simulink model "SIM_3DoF"  (R2024b)
settings: Solver=VariableStepAuto  StartTime=0.0  StopTime=300  RelTol=1e-6
values from neighbouring files (symbols this model uses):
  CL_zero = 0    [my_parameter_search.m]
  delta_maneuver = 1    [my_parameter_search.m]    (also in run_3DoF_SIM_SR22.m = 10; run_3DoF_SIM_SR22_Controller_Test.m = 0)
  deltaE = op_point.Inputs(1).u    [my_parameter_search.m]    (also in run_3DoF_SIM.m = -10; run_3DoF_SIM_SR22.m; run_3DoF_SIM_SR22_Controller_Test.m)
  gravity = 9.807    [run_3DoF_SIM.m]
  J = 30    [run_3DoF_SIM.m]
  M = M - 200    [my_parameter_search.m]
  p_maneuver = 1.5    [my_parameter_search.m]    (also in run_3DoF_SIM_SR22.m; run_3DoF_SIM_SR22_Controller_Test.m)
  rate_maneuver = 7    [my_parameter_search.m]    (also in run_3DoF_SIM_SR22.m; run_3DoF_SIM_SR22_Controller_Test.m)
  states_init = [0 op_point.States.x(2) op_point.States.x(3) op_point.States.x(4) 0 0]    [my_parameter_search.m]    (also in run_3DoF_SIM.m = [0 5000 0 80 0 0]; run_3DoF_SIM_SR22.m; run_3DoF_SIM_SR22_Controller_Test.m)
  t_maneuver = 0    [my_parameter_search.m]    (also in run_3DoF_SIM_SR22.m = 100; run_3DoF_SIM_SR22_Controller_Test.m)
  throttle = op_point.Inputs(2).u    [my_parameter_search.m]    (also in run_3DoF_SIM.m = 0.65; run_3DoF_SIM_SR22.m; run_3DoF_SIM_SR22_Controller_Test.m)
undefined symbols (not defined in the file or in its folder): CD_alpha, CL_alpha, CL_elev, CLEH_alpha, Cm_zero, Cw, down_wash, Sh, Sw, xa, xt
libraries: simulink_extras x7, aerolibatmos2 x2, slpidlib x2
(part 1 of 2)
settings Model: Creator=diego  LastModifiedBy=nicom

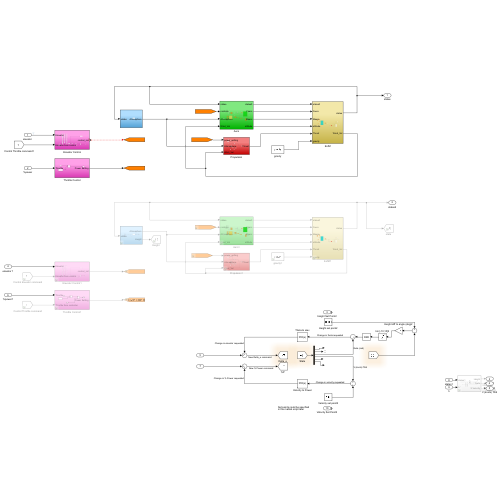
[thumbnail: Simulink's stored preview of the top-level diagram]
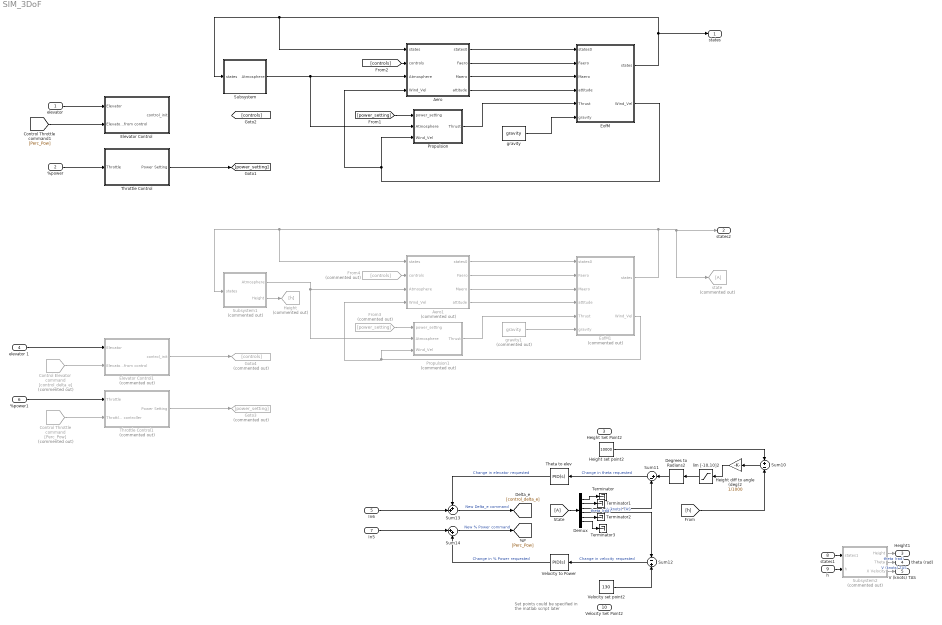
== system SIM_3DoF ==
  note: Set points could be specified in the matlab script later
  "elevator " : Inport
  %power : Inport  Port=2
  Height Set Point2 : Inport  Port=3
  elevator 1 : Inport  Port=4
  In6 : Inport  Port=5
  %power1 : Inport  Port=6
  In5 : Inport  Port=7
  states1 : Inport  Port=8
  h : Inport  Port=9
  Velocity Set Point2 : Inport  Port=10
  Aero : Subsystem
  Aero1 : Subsystem  Commented=on
  Control Elevator command : From  Commented=on  GotoTag=control_delta_e
  Control Throttle command : From  Commented=on  GotoTag=Perc_Pow
  Degrees to Radians2 : simulink_extras/Transformations/Degrees to Radians
  Demux : Demux  Outputs=6
  Elevator Control : Subsystem
  Elevator Control1 : Subsystem  Commented=on
  EofM : Subsystem
  EofM1 : Subsystem  Commented=on
  From3 : From  Commented=on  GotoTag=power_setting
  From4 : From  Commented=on  GotoTag=controls
  Goto3 : Goto  Commented=on  GotoTag=power_setting
  Goto4 : Goto  Commented=on  GotoTag=controls
  Height : Goto  Commented=on  GotoTag=h
  Height diff to angle (deg)2 : Gain  Gain=1/1000
  Height set point2 : Constant  Value=10000
  Propulsion : Subsystem
  Propulsion1 : Subsystem  Commented=on
  State : From
  Subsystem : Subsystem
  Subsystem1 : Subsystem  Commented=on
  Subsystem2 : Subsystem  Commented=on
  Sum10 : Sum  Inputs=+|-
  Sum11 : Sum  Inputs=|+-
  Sum12 : Sum  Inputs=-|+
  Sum13 : Sum  Inputs=++|
  Sum14 : Sum  Inputs=|++
  Terminator{,1..3} (4 alike) : Terminator
  Theta to elev : slpidlib/PID Controller  Controller=PID  Form=Parallel  TimeDomain=Continuous-time  UseExternalTs=off  SampleTime=-1  IntegratorMethod=Forward Euler  FilterMethod=Forward Euler  ControllerParametersSource=internal  P=1  I=1  UseKiTs=off  D=0  UseExternalDerivativeSource=off  N=100  UseFilter=on  TunerSelectOption=Transfer Function Based (PID Tuner App)  InitialConditionSource=internal  InitialConditionForIntegrator=0  InitialConditionForFilter=0  DifferentiatorICPrevScaledInput=0  ExternalReset=none  TrackingMode=off  Kt=1  LimitOutput=off  SatLimitsSource=internal  UpperSaturationLimit=inf  LowerSaturationLimit=-inf  LinearizeAsGain=on  AntiWindupMode=none  Kb=1  LimitIntegrator=off  UpperIntegratorSaturationLimit=inf  LowerIntegratorSaturationLimit=-inf  POutMin=[]  POutMax=[]  IOutMin=[]  IOutMax=[]  DOutMin=[]  DOutMax=[]  NOutMin=[]  NOutMax=[]  SumOutMin=[]  SumOutMax=[]  SaturationOutMin=[]  SaturationOutMax=[]  PParamMin=[]  PParamMax=[]  IParamMin=[]  IParamMax=[]  DParamMin=[]  DParamMax=[]  NParamMin=[]  NParamMax=[]  KbParamMin=[]  KbParamMax=[]  KtParamMin=[]  KtParamMax=[]  KbOutMin=[]  KbOutMax=[]  KtOutMin=[]  KtOutMax=[]  IntegratorOutMin=[]  IntegratorOutMax=[]  FilterOutMin=[]  FilterOutMax=[]  SumI1OutMin=[]  SumI1OutMax=[]  SumI2OutMin=[]  SumI2OutMax=[]  SumI3OutMin=[]  SumI3OutMax=[]  SumI4OutMin=[]  SumI4OutMax=[]  SumDOutMin=[]  SumDOutMax=[]  DifferentiatorOutMin=[]  DifferentiatorOutMax=[]  FilterDiffOutCoefMin=[]  FilterDiffOutCoefMax=[]  ReciprocalOutMin=[]  ReciprocalOutMax=[]  SumDenOutMin=[]  SumDenOutMax=[]  SumNumOutMin=[]  SumNumOutMax=[]  DivideOutMin=[]  DivideOutMax=[]  UdiffTsProdOutMin=[]  UdiffTsProdOutMax=[]  NTsProdOutMin=[]  NTsProdOutMax=[]  UintegralTsProdOutMin=[]  UintegralTsProdOutMax=[]  UngainTsProdOutMin=[]  UngainTsProdOutMax=[]  ClampingZeroOutDataTypeStr=Inherit: Inherit via back propagation  ClampingZeroOutMin=[]  ClampingZeroOutMax=[]  FilterDenConstantOutDataTypeStr=Inherit: Inherit via back propagation  FilterDenConstantOutMin=[]  FilterDenConstantOutMax=[]  PCopyOutDataTypeStr=Inherit: Inherit via back propagation  PCopyOutMin=[]  PCopyOutMax=[]  NCopyOutDataTypeStr=Inherit: Inherit via back propagation  NCopyOutMin=[]  NCopyOutMax=[]  IntegratorContinuousStateAttributes=''  IntegratorStateMustResolveToSignalObject=off  IntegratorRTWStateStorageClass=Auto  FilterContinuousStateAttributes=''  FilterStateMustResolveToSignalObject=off  FilterRTWStateStorageClass=Auto  ParallelPVariant=InternalParameters  IdealPVariant=Disabled  IVariant=InternalParameters  DVariant=InternalParameters  IntegratorVariant=Continuous  SatVariant=Disabled  AWVariant=Passthrough  PCopyVariant=Disabled  TRVariant=Disabled  FdbkBlocksVariant=Forward  IdealPFdbkVariant=Disabled  SatFdbkVariant=Disabled  DerivativeFilterVariant=ContFilter  NVariant=InternalParameters  NCopyVariant=Disabled  FilterICVariant=InternalICsFilter  IntegratorICVariant=InternalICs  ExternalResetVariant=Disabled  TRSumVariant=Passthrough  SumFdbkVariant=Disabled  SumVariant=Sum_PID  TsampFilterVariant=InternalTs  TsampNgainVariant=Passthrough  TsampIntegralVariant=Disabled_SignalSpec  ExternalSaturationOutDataTypeStr=Inherit: Same as second input  DerivativeSourceVariant=ErrorSignal  PreIntVariant=InternalPreInt
  Throttle Control : Subsystem
  Throttle Control1 : Subsystem  Commented=on
  Velocity set point2 : Constant  Value=130
  Velocity to Power : slpidlib/PID Controller  Controller=PID  Form=Parallel  TimeDomain=Continuous-time  UseExternalTs=off  SampleTime=-1  IntegratorMethod=Forward Euler  FilterMethod=Forward Euler  ControllerParametersSource=internal  P=1  I=1  UseKiTs=off  D=0  UseExternalDerivativeSource=off  N=100  UseFilter=on  TunerSelectOption=Transfer Function Based (PID Tuner App)  InitialConditionSource=internal  InitialConditionForIntegrator=0  InitialConditionForFilter=0  DifferentiatorICPrevScaledInput=0  ExternalReset=none  TrackingMode=off  Kt=1  LimitOutput=off  SatLimitsSource=internal  UpperSaturationLimit=inf  LowerSaturationLimit=-inf  LinearizeAsGain=on  AntiWindupMode=none  Kb=1  LimitIntegrator=off  UpperIntegratorSaturationLimit=inf  LowerIntegratorSaturationLimit=-inf  POutMin=[]  POutMax=[]  IOutMin=[]  IOutMax=[]  DOutMin=[]  DOutMax=[]  NOutMin=[]  NOutMax=[]  SumOutMin=[]  SumOutMax=[]  SaturationOutMin=[]  SaturationOutMax=[]  PParamMin=[]  PParamMax=[]  IParamMin=[]  IParamMax=[]  DParamMin=[]  DParamMax=[]  NParamMin=[]  NParamMax=[]  KbParamMin=[]  KbParamMax=[]  KtParamMin=[]  KtParamMax=[]  KbOutMin=[]  KbOutMax=[]  KtOutMin=[]  KtOutMax=[]  IntegratorOutMin=[]  IntegratorOutMax=[]  FilterOutMin=[]  FilterOutMax=[]  SumI1OutMin=[]  SumI1OutMax=[]  SumI2OutMin=[]  SumI2OutMax=[]  SumI3OutMin=[]  SumI3OutMax=[]  SumI4OutMin=[]  SumI4OutMax=[]  SumDOutMin=[]  SumDOutMax=[]  DifferentiatorOutMin=[]  DifferentiatorOutMax=[]  FilterDiffOutCoefMin=[]  FilterDiffOutCoefMax=[]  ReciprocalOutMin=[]  ReciprocalOutMax=[]  SumDenOutMin=[]  SumDenOutMax=[]  SumNumOutMin=[]  SumNumOutMax=[]  DivideOutMin=[]  DivideOutMax=[]  UdiffTsProdOutMin=[]  UdiffTsProdOutMax=[]  NTsProdOutMin=[]  NTsProdOutMax=[]  UintegralTsProdOutMin=[]  UintegralTsProdOutMax=[]  UngainTsProdOutMin=[]  UngainTsProdOutMax=[]  ClampingZeroOutDataTypeStr=Inherit: Inherit via back propagation  ClampingZeroOutMin=[]  ClampingZeroOutMax=[]  FilterDenConstantOutDataTypeStr=Inherit: Inherit via back propagation  FilterDenConstantOutMin=[]  FilterDenConstantOutMax=[]  PCopyOutDataTypeStr=Inherit: Inherit via back propagation  PCopyOutMin=[]  PCopyOutMax=[]  NCopyOutDataTypeStr=Inherit: Inherit via back propagation  NCopyOutMin=[]  NCopyOutMax=[]  IntegratorContinuousStateAttributes=''  IntegratorStateMustResolveToSignalObject=off  IntegratorRTWStateStorageClass=Auto  FilterContinuousStateAttributes=''  FilterStateMustResolveToSignalObject=off  FilterRTWStateStorageClass=Auto  ParallelPVariant=InternalParameters  IdealPVariant=Disabled  IVariant=InternalParameters  DVariant=InternalParameters  IntegratorVariant=Continuous  SatVariant=Disabled  AWVariant=Passthrough  PCopyVariant=Disabled  TRVariant=Disabled  FdbkBlocksVariant=Forward  IdealPFdbkVariant=Disabled  SatFdbkVariant=Disabled  DerivativeFilterVariant=ContFilter  NVariant=InternalParameters  NCopyVariant=Disabled  FilterICVariant=InternalICsFilter  IntegratorICVariant=InternalICs  ExternalResetVariant=Disabled  TRSumVariant=Passthrough  SumFdbkVariant=Disabled  SumVariant=Sum_PID  TsampFilterVariant=InternalTs  TsampNgainVariant=Passthrough  TsampIntegralVariant=Disabled_SignalSpec  ExternalSaturationOutDataTypeStr=Inherit: Same as second input  DerivativeSourceVariant=ErrorSignal  PreIntVariant=InternalPreInt
  gravity : Constant  Value=gravity
  gravity1 : Constant  Commented=on  Value=gravity
  lim [-10,10]2 : Saturate  UpperLimit=10  LowerLimit=-10
  state : Goto  Commented=on
  states : Outport
  states2 : Outport  Port=2
  Height1 : Outport  Port=3
  theta (rad) : Outport  Port=4
  V (knots) TAS : Outport  Port=5
  wires:
  Aero/2(Faero) -> EofM/2(Faero)
  Aero/3(Maero) -> EofM/3(Maero)
  EofM/1(states) -> states/1, Subsystem/1(states), Aero/1(states)
  Subsystem/1(Atmosphere) -> Aero/3(Atmosphere), Propulsion/2(Atmosphere)
  EofM/2(Wind_Vel) -> Propulsion/3(Wind_Vel), Aero/4(Wind_Vel)
  Aero/1(states0) -> EofM/1(states0)
  [controls] -> Aero/2(controls)
  [power_setting] -> Propulsion/1("power_setting ")
  ? -> [controls]
  Aero/4(attitude) -> EofM/4(attitude)
  gravity/1 -> EofM/6(gravity)
  Propulsion/1(Thrust) -> EofM/5(Thrust)
  "elevator "/1 -> Elevator Control/1(Elevator)
  %power/1 -> Throttle Control/1(Throttle)
  Throttle Control/1(Power Setting) -> [power_setting]
  elevator 1/1 -> Elevator Control1/1(Elevator)
  Velocity set point2/1 -> Sum12/2
  Subsystem1/2(Height) -> Height/1
  Throttle Control1/1(Power Setting) -> Goto3/1
  Aero1/3(Maero) -> EofM1/3(Maero)
  From4/1 -> Aero1/2(controls)
  Aero1/2(Faero) -> EofM1/2(Faero)
  Subsystem2/2(Theta) -> theta (rad)/1  "theta (rad)"
  Demux/2 -> Terminator1/1
  gravity1/1 -> EofM1/6(gravity)
  Aero1/1(states0) -> EofM1/1(states0)
  h/1 -> Subsystem2/2(h)
  In5/1 -> Sum14/1
  states1/1 -> Subsystem2/1(states1)
  Sum10/1 -> Height diff to angle (deg)2/1
  %power1/1 -> Throttle Control1/1(Throttle)
  State/1 -> Demux/1
  Demux/6 -> Terminator3/1
  Height set point2/1 -> Sum10/1
  Theta to elev/1 -> Sum13/1  "Change in elevator requested"
  Demux/4 -> Sum12/1  "V (knots) TAS"
  Subsystem2/1(Height) -> Height1/1
  Sum12/1 -> Velocity to Power/1  "Change in velocity requested"
  Control Elevator command/1 -> Elevator Control1/2(Elevator from control)
  Elevator Control1/1(control_init) -> Goto4/1
  lim [-10,10]2/1 -> Degrees to Radians2/1
  EofM1/1(states) -> states2/1, state/1, Subsystem1/1(states), Aero1/1(states)
  Demux/1 -> Terminator/1
  Velocity to Power/1 -> Sum14/2  "Change in % Power requested"
  Demux/3 -> Sum11/2  "theta (rad)"
  Sum13/1 -> [control_delta_e]  "New Delta_e command"
  [h] -> Sum10/2
  Degrees to Radians2/1 -> Sum11/1
  Control Throttle command/1 -> Throttle Control1/2(Throttle from controller)
  EofM1/2(Wind_Vel) -> Aero1/4(Wind_Vel), Propulsion1/3(Wind_Vel)
  Subsystem1/1(Atmosphere) -> Aero1/3(Atmosphere), Propulsion1/2(Atmosphere)
  From3/1 -> Propulsion1/1("power_setting ")
  Sum14/1 -> [Perc_Pow]  "New % Power command"
  Sum11/1 -> Theta to elev/1  "Change in theta requested"
  In6/1 -> Sum13/2
  Demux/5 -> Terminator2/1
  Subsystem2/3(X Velocity) -> V (knots) TAS/1  "V (knots) TAS"
  Propulsion1/1(Thrust) -> EofM1/5(Thrust)
  Aero1/4(attitude) -> EofM1/4(attitude)
  Height diff to angle (deg)2/1 -> lim [-10,10]2/1
  [Perc_Pow] -> Elevator Control/2(Elevator from control)

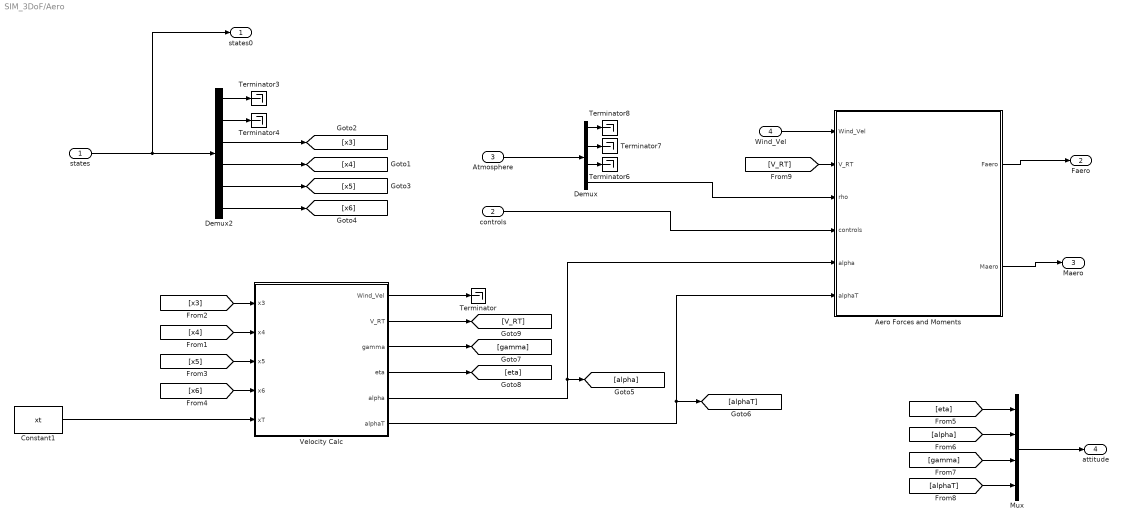
== system SIM_3DoF/Aero ==
  states : Inport
  controls : Inport  Port=2
  Atmosphere : Inport  Port=3
  Wind_Vel : Inport  Port=4
  Aero Forces and Moments : Subsystem
  Constant1 : Constant  Value=xt
  Demux : Demux
  Demux2 : Demux  Outputs=6
  Mux : Mux
  Terminator{,3..4,6..8} (6 alike) : Terminator
  Velocity Calc : Subsystem
  states0 : Outport
  Faero : Outport  Port=2
  Maero : Outport  Port=3
  attitude : Outport  Port=4
  wires:
  Atmosphere/1 -> Demux/1
  states/1 -> Demux2/1, states0/1
  Wind_Vel/1 -> Aero Forces and Moments/1(Wind_Vel)
  Demux/4 -> Aero Forces and Moments/3(rho)
  Aero Forces and Moments/1(Faero) -> Faero/1
  Aero Forces and Moments/2(Maero) -> Maero/1
  controls/1 -> Aero Forces and Moments/4(controls)
  Constant1/1 -> Velocity Calc/5(xT)
  Velocity Calc/4(eta) -> [eta]
  Velocity Calc/1(Wind_Vel) -> Terminator/1
  Velocity Calc/3(gamma) -> [gamma]
  Demux2/1 -> Terminator3/1
  Demux2/2 -> Terminator4/1
  Demux2/3 -> [x3]
  Demux2/4 -> [x4]
  Demux2/5 -> [x5]
  Demux2/6 -> [x6]
  Demux/1 -> Terminator8/1
  Demux/2 -> Terminator7/1
  Demux/3 -> Terminator6/1
  Velocity Calc/5(alpha) -> Aero Forces and Moments/5(alpha), [alpha]
  Velocity Calc/6(alphaT) -> Aero Forces and Moments/6(alphaT), [alphaT]
  [x3] -> Velocity Calc/1(x3)
  [x4] -> Velocity Calc/2(x4)
  [x6] -> Velocity Calc/4(x6)
  [x5] -> Velocity Calc/3(x5)
  Mux/1 -> attitude/1
  [eta] -> Mux/1
  [alpha] -> Mux/2
  [gamma] -> Mux/3
  [alphaT] -> Mux/4
  Velocity Calc/2(V_RT) -> [V_RT]
  [V_RT] -> Aero Forces and Moments/2(V_RT)

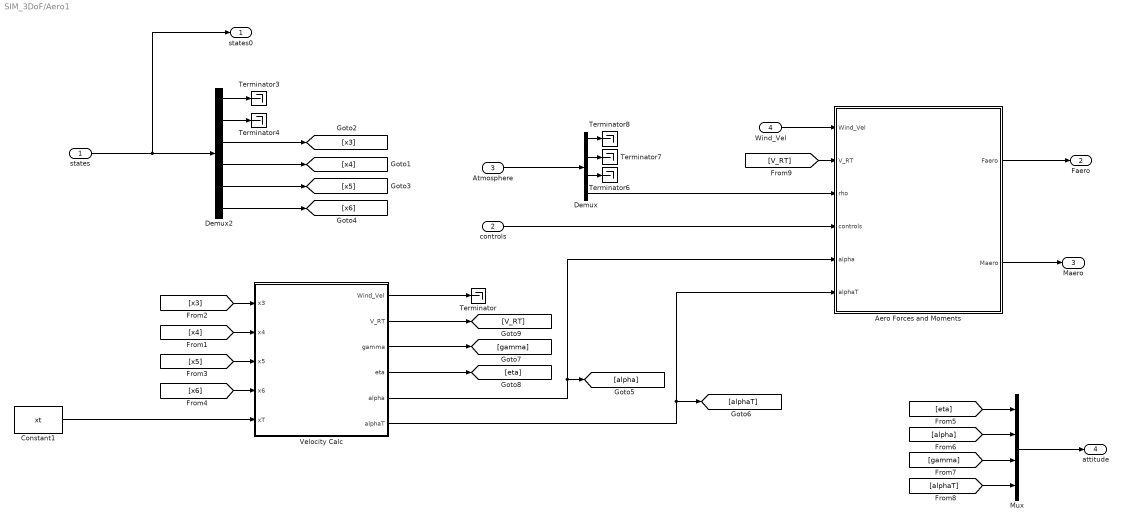
== system SIM_3DoF/Aero1 ==
  states : Inport
  controls : Inport  Port=2
  Atmosphere : Inport  Port=3
  Wind_Vel : Inport  Port=4
  Aero Forces and Moments : Subsystem
  Constant1 : Constant  Value=xt
  Demux : Demux
  Demux2 : Demux  Outputs=6
  Mux : Mux
  Terminator{,3..4,6..8} (6 alike) : Terminator
  Velocity Calc : Subsystem
  states0 : Outport
  Faero : Outport  Port=2
  Maero : Outport  Port=3
  attitude : Outport  Port=4
  wires:
  Atmosphere/1 -> Demux/1
  states/1 -> Demux2/1, states0/1
  Wind_Vel/1 -> Aero Forces and Moments/1(Wind_Vel)
  Demux/4 -> Aero Forces and Moments/3(rho)
  Aero Forces and Moments/1(Faero) -> Faero/1
  Aero Forces and Moments/2(Maero) -> Maero/1
  controls/1 -> Aero Forces and Moments/4(controls)
  Constant1/1 -> Velocity Calc/5(xT)
  Velocity Calc/4(eta) -> [eta]
  Velocity Calc/1(Wind_Vel) -> Terminator/1
  Velocity Calc/3(gamma) -> [gamma]
  Demux2/1 -> Terminator3/1
  Demux2/2 -> Terminator4/1
  Demux2/3 -> [x3]
  Demux2/4 -> [x4]
  Demux2/5 -> [x5]
  Demux2/6 -> [x6]
  Demux/1 -> Terminator8/1
  Demux/2 -> Terminator7/1
  Demux/3 -> Terminator6/1
  Velocity Calc/5(alpha) -> Aero Forces and Moments/5(alpha), [alpha]
  Velocity Calc/6(alphaT) -> Aero Forces and Moments/6(alphaT), [alphaT]
  [x3] -> Velocity Calc/1(x3)
  [x4] -> Velocity Calc/2(x4)
  [x6] -> Velocity Calc/4(x6)
  [x5] -> Velocity Calc/3(x5)
  Mux/1 -> attitude/1
  [eta] -> Mux/1
  [alpha] -> Mux/2
  [gamma] -> Mux/3
  [alphaT] -> Mux/4
  Velocity Calc/2(V_RT) -> [V_RT]
  [V_RT] -> Aero Forces and Moments/2(V_RT)

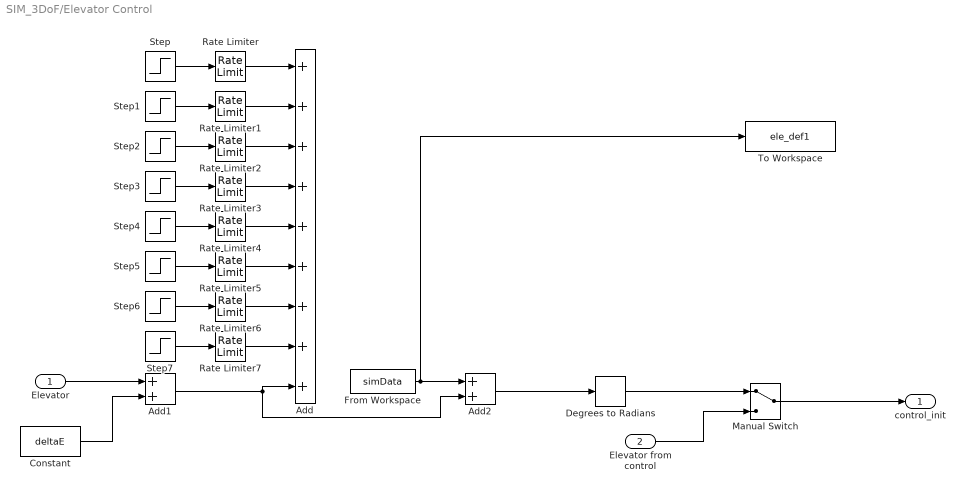
== system SIM_3DoF/Elevator Control ==
  Elevator : Inport
  Elevator from control : Inport  Port=2
  Add : Sum  Inputs=+++++++++
  Add1 : Sum
  Add2 : Sum
  Constant : Constant  Value=deltaE
  Degrees to Radians : simulink_extras/Transformations/Degrees to Radians
  From Workspace : FromWorkspace  VariableName=simData  Interpolate=off  OutputAfterFinalValue=Setting to zero
  Manual Switch : ManualSwitch
  Rate Limiter{,1..7} (8 alike) : RateLimiter  RisingSlewLimit=rate_maneuver  FallingSlewLimit=-rate_maneuver  SampleTimeMode=inherited
  Step : Step  Time=t_maneuver  After=delta_maneuver  SampleTime=0
  Step1 : Step  Time=t_maneuver+3*p_maneuver  After=-delta_maneuver  SampleTime=0
  Step2 : Step  Time=t_maneuver+3*p_maneuver  After=-delta_maneuver  SampleTime=0
  Step3 : Step  Time=t_maneuver+5*p_maneuver  After=delta_maneuver  SampleTime=0
  Step4 : Step  Time=t_maneuver+5*p_maneuver  After=delta_maneuver  SampleTime=0
  Step5 : Step  Time=t_maneuver+6*p_maneuver  After=-delta_maneuver  SampleTime=0
  Step6 : Step  Time=t_maneuver+6*p_maneuver  After=-delta_maneuver  SampleTime=0
  Step7 : Step  Time=t_maneuver+7*p_maneuver  After=delta_maneuver  SampleTime=0
  To Workspace : ToWorkspace  VariableName=ele_def1  SampleTime=-1
  control_init : Outport
  wires:
  Add1/1 -> Add2/2, Add/9
  Step1/1 -> Rate Limiter1/1
  Rate Limiter3/1 -> Add/4
  Add2/1 -> Degrees to Radians/1
  Step6/1 -> Rate Limiter6/1
  Constant/1 -> Add1/2
  Rate Limiter1/1 -> Add/2
  Rate Limiter4/1 -> Add/5
  Step2/1 -> Rate Limiter2/1
  From Workspace/1 -> Add2/1, To Workspace/1
  Elevator from control/1 -> Manual Switch/2
  Rate Limiter7/1 -> Add/8
  Rate Limiter5/1 -> Add/6
  Step3/1 -> Rate Limiter3/1
  Rate Limiter/1 -> Add/1
  Rate Limiter6/1 -> Add/7
  Step5/1 -> Rate Limiter5/1
  Manual Switch/1 -> control_init/1
  Step/1 -> Rate Limiter/1
  Degrees to Radians/1 -> Manual Switch/1
  Step7/1 -> Rate Limiter7/1
  Elevator/1 -> Add1/1
  Rate Limiter2/1 -> Add/3
  Step4/1 -> Rate Limiter4/1

== system SIM_3DoF/Elevator Control1 ==
  Elevator : Inport
  Elevator from control : Inport  Port=2
  Add : Sum  Commented=on  Inputs=+++++++++
  Add1 : Sum  Commented=on
  Add2 : Sum  Commented=on
  Constant : Constant  Commented=on  Value=deltaE
  Degrees to Radians : simulink_extras/Transformations/Degrees to Radians  Commented=on
  From Workspace : FromWorkspace  Commented=on  VariableName=simData  Interpolate=off  OutputAfterFinalValue=Setting to zero
  Manual Switch : ManualSwitch
  Rate Limiter{,1..7} (8 alike) : RateLimiter  Commented=on  RisingSlewLimit=rate_maneuver  FallingSlewLimit=-rate_maneuver  SampleTimeMode=inherited
  Step : Step  Commented=on  Time=t_maneuver  After=delta_maneuver  SampleTime=0
  Step1 : Step  Commented=on  Time=t_maneuver+3*p_maneuver  After=-delta_maneuver  SampleTime=0
  Step2 : Step  Commented=on  Time=t_maneuver+3*p_maneuver  After=-delta_maneuver  SampleTime=0
  Step3 : Step  Commented=on  Time=t_maneuver+5*p_maneuver  After=delta_maneuver  SampleTime=0
  Step4 : Step  Commented=on  Time=t_maneuver+5*p_maneuver  After=delta_maneuver  SampleTime=0
  Step5 : Step  Commented=on  Time=t_maneuver+6*p_maneuver  After=-delta_maneuver  SampleTime=0
  Step6 : Step  Commented=on  Time=t_maneuver+6*p_maneuver  After=-delta_maneuver  SampleTime=0
  Step7 : Step  Commented=on  Time=t_maneuver+7*p_maneuver  After=delta_maneuver  SampleTime=0
  To Workspace : ToWorkspace  Commented=on  VariableName=ele_def  SampleTime=-1
  control_init : Outport
  wires:
  Step/1 -> Rate Limiter/1
  Step1/1 -> Rate Limiter1/1
  Step2/1 -> Rate Limiter2/1
  Step3/1 -> Rate Limiter3/1
  Step4/1 -> Rate Limiter4/1
  Step5/1 -> Rate Limiter5/1
  Step6/1 -> Rate Limiter6/1
  Step7/1 -> Rate Limiter7/1
  Rate Limiter/1 -> Add/1
  Rate Limiter1/1 -> Add/2
  Rate Limiter2/1 -> Add/3
  Rate Limiter3/1 -> Add/4
  Rate Limiter4/1 -> Add/5
  Rate Limiter5/1 -> Add/6
  Rate Limiter6/1 -> Add/7
  Rate Limiter7/1 -> Add/8
  Elevator/1 -> Add1/1
  Add1/1 -> Add2/2, Add/9
  Constant/1 -> Add1/2
  From Workspace/1 -> Add2/1, To Workspace/1
  Add2/1 -> Degrees to Radians/1
  Elevator from control/1 -> Manual Switch/2
  Degrees to Radians/1 -> Manual Switch/1
  Manual Switch/1 -> control_init/1

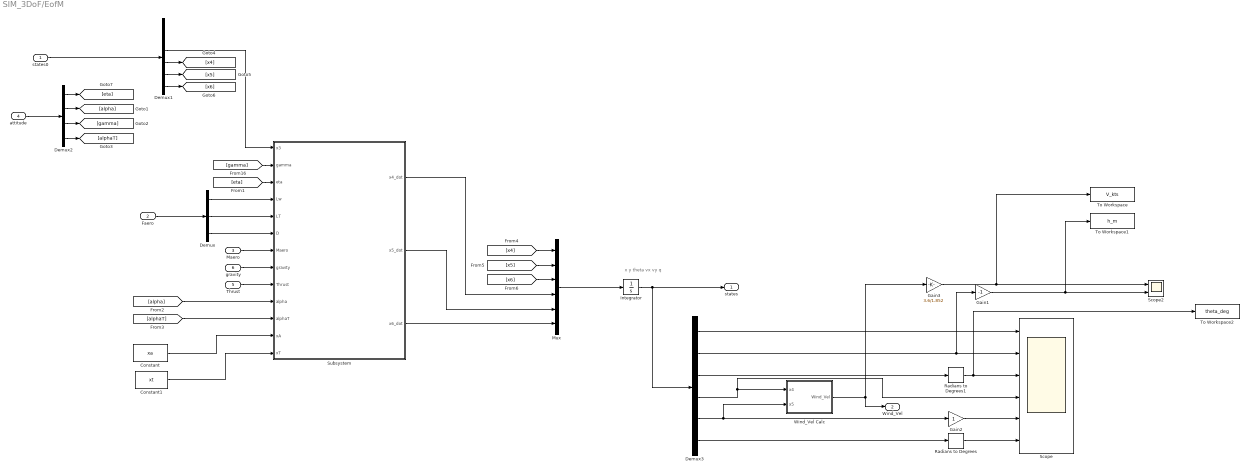
== system SIM_3DoF/EofM ==
  note: x y theta vx vy q
  states0 : Inport
  Faero : Inport  Port=2
  Maero : Inport  Port=3
  attitude : Inport  Port=4
  Thrust : Inport  Port=5
  gravity : Inport  Port=6
  Constant : Constant  Value=xa
  Constant1 : Constant  Value=xt
  Demux : Demux  Outputs=3
  Demux1 : Demux  Outputs=6
  Demux2 : Demux
  Demux3 : Demux  Outputs=6
  Gain1 : Gain  Gain=-1
  Gain2 : Gain
  Gain3 : Gain  Gain=3.6/1.852
  Integrator : Integrator  InitialCondition=states_init
  Mux : Mux  Inputs=6
  Radians to Degrees : simulink_extras/Transformations/Radians to Degrees
  Radians to Degrees1 : simulink_extras/Transformations/Radians to Degrees
  Scope : Scope  NumInputPorts=6
  Scope2 : Scope  NumInputPorts=2
  Subsystem : Subsystem
  To Workspace : ToWorkspace  VariableName=V_kts  SampleTime=-1
  To Workspace1 : ToWorkspace  VariableName=h_m  SampleTime=-1
  To Workspace2 : ToWorkspace  VariableName=theta_deg  SampleTime=-1
  Wind_Vel Calc : Subsystem
  states : Outport
  Wind_Vel : Outport  Port=2
  wires:
  Integrator/1 -> states/1, Demux3/1
  Mux/1 -> Integrator/1
  Faero/1 -> Demux/1
  Demux/1 -> Subsystem/4(Lw)
  Demux/2 -> Subsystem/5(LT)
  Demux/3 -> Subsystem/6(D)
  Maero/1 -> Subsystem/7(Maero)
  gravity/1 -> Subsystem/8(gravity)
  Thrust/1 -> Subsystem/9(Thrust)
  Subsystem/1(x4_dot) -> Mux/4
  Subsystem/2(x5_dot) -> Mux/5
  Subsystem/3(x6_dot) -> Mux/6
  Wind_Vel Calc/1(Wind_Vel) -> Gain3/1, Wind_Vel/1
  attitude/1 -> Demux2/1
  Demux2/1 -> [eta]
  Demux2/2 -> [alpha]
  Demux2/3 -> [gamma]
  Demux2/4 -> [alphaT]
  [eta] -> Subsystem/3(eta)
  [gamma] -> Subsystem/2(gamma)
  [alpha] -> Subsystem/10(alpha)
  [alphaT] -> Subsystem/11(alphaT)
  Demux1/3 -> Subsystem/1(x3)
  Demux1/4 -> [x4]
  Demux1/5 -> [x5]
  Demux1/6 -> [x6]
  [x4] -> Mux/1
  [x5] -> Mux/2
  [x6] -> Mux/3
  Demux3/5 -> Wind_Vel Calc/2(x5), Gain2/1
  Demux3/4 -> Scope/4, Wind_Vel Calc/1(x4)
  Demux3/1 -> Scope/1
  Demux3/3 -> Radians to Degrees1/1
  Demux3/6 -> Radians to Degrees/1
  states0/1 -> Demux1/1
  Constant/1 -> Subsystem/12("xA ")
  Constant1/1 -> Subsystem/13(xT)
  Radians to Degrees/1 -> Scope/6
  Radians to Degrees1/1 -> Scope/3, To Workspace2/1
  Gain2/1 -> Scope/5
  Demux3/2 -> Gain1/1, Scope/2
  Gain1/1 -> To Workspace1/1, Scope2/2
  Gain3/1 -> To Workspace/1, Scope2/1

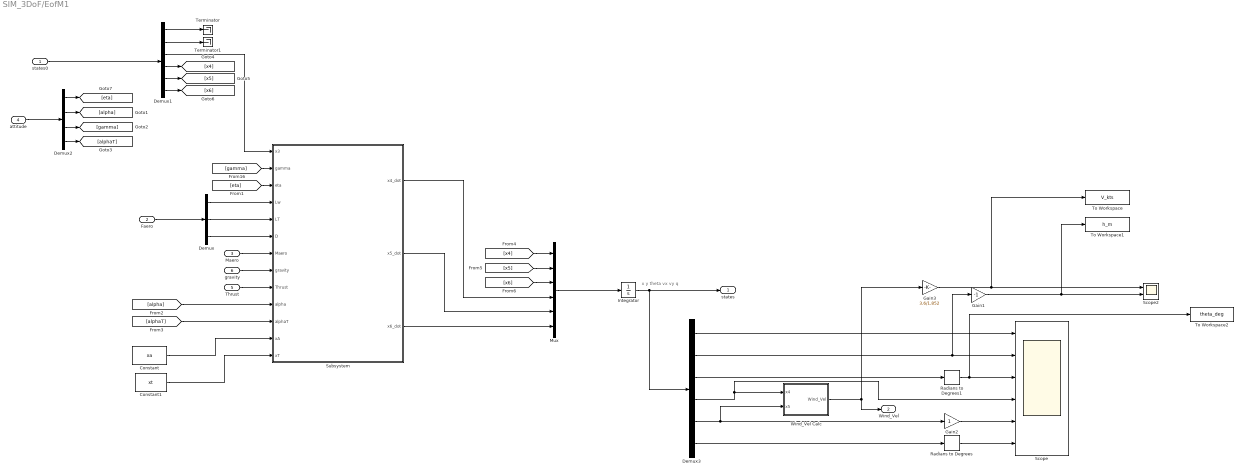
== system SIM_3DoF/EofM1 ==
  note: x y theta vx vy q
  states0 : Inport
  Faero : Inport  Port=2
  Maero : Inport  Port=3
  attitude : Inport  Port=4
  Thrust : Inport  Port=5
  gravity : Inport  Port=6
  Constant : Constant  Value=xa
  Constant1 : Constant  Value=xt
  Demux : Demux  Outputs=3
  Demux1 : Demux  Outputs=6
  Demux2 : Demux
  Demux3 : Demux  Outputs=6
  Gain1 : Gain  Gain=-1
  Gain2 : Gain
  Gain3 : Gain  Gain=3.6/1.852
  Integrator : Integrator  InitialCondition=states_init
  Mux : Mux  Inputs=6
  Radians to Degrees : simulink_extras/Transformations/Radians to Degrees
  Radians to Degrees1 : simulink_extras/Transformations/Radians to Degrees
  Scope : Scope  NumInputPorts=6
  Scope2 : Scope  NumInputPorts=2
  Subsystem : Subsystem
  Terminator : Terminator
  Terminator1 : Terminator
  To Workspace : ToWorkspace  VariableName=V_kts  SampleTime=-1
  To Workspace1 : ToWorkspace  VariableName=h_m  SampleTime=-1
  To Workspace2 : ToWorkspace  VariableName=theta_deg  SampleTime=-1
  Wind_Vel Calc : Subsystem
  states : Outport
  Wind_Vel : Outport  Port=2
  wires:
  Integrator/1 -> states/1, Demux3/1
  Mux/1 -> Integrator/1
  Faero/1 -> Demux/1
  Demux/1 -> Subsystem/4(Lw)
  Demux/2 -> Subsystem/5(LT)
  Demux/3 -> Subsystem/6(D)
  Maero/1 -> Subsystem/7(Maero)
  gravity/1 -> Subsystem/8(gravity)
  Thrust/1 -> Subsystem/9(Thrust)
  Subsystem/1(x4_dot) -> Mux/4
  Subsystem/2(x5_dot) -> Mux/5
  Subsystem/3(x6_dot) -> Mux/6
  Wind_Vel Calc/1(Wind_Vel) -> Gain3/1, Wind_Vel/1
  attitude/1 -> Demux2/1
  Demux2/1 -> [eta]
  Demux2/2 -> [alpha]
  Demux2/3 -> [gamma]
  Demux2/4 -> [alphaT]
  [eta] -> Subsystem/3(eta)
  [gamma] -> Subsystem/2(gamma)
  [alpha] -> Subsystem/10(alpha)
  [alphaT] -> Subsystem/11(alphaT)
  Demux1/3 -> Subsystem/1(x3)
  Demux1/4 -> [x4]
  Demux1/5 -> [x5]
  Demux1/6 -> [x6]
  [x4] -> Mux/1
  [x5] -> Mux/2
  [x6] -> Mux/3
  Demux3/5 -> Wind_Vel Calc/2(x5), Gain2/1
  Demux3/4 -> Scope/4, Wind_Vel Calc/1(x4)
  Demux3/1 -> Scope/1
  Demux3/3 -> Radians to Degrees1/1
  Demux3/6 -> Radians to Degrees/1
  states0/1 -> Demux1/1
  Constant/1 -> Subsystem/12("xA ")
  Constant1/1 -> Subsystem/13(xT)
  Radians to Degrees/1 -> Scope/6
  Radians to Degrees1/1 -> Scope/3, To Workspace2/1
  Gain2/1 -> Scope/5
  Demux3/2 -> Gain1/1, Scope/2
  Gain1/1 -> To Workspace1/1, Scope2/2
  Gain3/1 -> To Workspace/1, Scope2/1
  Demux1/1 -> Terminator/1
  Demux1/2 -> Terminator1/1

== system SIM_3DoF/Propulsion ==
  "power_setting " : Inport
  Atmosphere : Inport  Port=2
  Wind_Vel : Inport  Port=3
  Demux : Demux
  Divide : Product  Inputs=*/
  Divide1 : Product  Inputs=*/
  Dot Product : DotProduct  OutDataTypeStr=Inherit: Inherit via internal rule
  Dot Product2 : DotProduct  OutDataTypeStr=Inherit: Inherit via internal rule
  Exp : Math  Operator=pow
  Power - W (315hp) : Constant  Value=234895
  Terminator : Terminator
  Terminator1 : Terminator
  Terminator2 : Terminator
  eta_p : Constant  Value=0.75
  n : Constant  Value=0.7
  rho0 : Constant  Value=1.225
  Thrust : Outport
  wires:
  "power_setting "/1 -> Dot Product/2
  Atmosphere/1 -> Demux/1
  Demux/4 -> Divide/1
  rho0/1 -> Divide/2
  Divide/1 -> Exp/1
  n/1 -> Exp/2
  Divide1/1 -> Thrust/1
  Wind_Vel/1 -> Divide1/2
  Dot Product2/1 -> Dot Product/1
  Power - W (315hp)/1 -> Dot Product2/2
  eta_p/1 -> Dot Product2/1
  Demux/1 -> Terminator/1
  Demux/2 -> Terminator1/1
  Demux/3 -> Terminator2/1
  Dot Product/1 -> Divide1/1

== system SIM_3DoF/Propulsion1 ==
  "power_setting " : Inport
  Atmosphere : Inport  Port=2
  Wind_Vel : Inport  Port=3
  Demux : Demux
  Divide : Product  Inputs=*/
  Divide1 : Product  Inputs=*/
  Dot Product : DotProduct  OutDataTypeStr=Inherit: Inherit via internal rule
  Dot Product2 : DotProduct  OutDataTypeStr=Inherit: Inherit via internal rule
  Exp : Math  Operator=pow
  Power - W (315hp) : Constant  Value=234895
  Terminator : Terminator
  Terminator1 : Terminator
  Terminator2 : Terminator
  eta_p : Constant  Value=0.75
  n : Constant  Value=0.7
  rho0 : Constant  Value=1.225
  Thrust : Outport
  wires:
  "power_setting "/1 -> Dot Product/2
  Atmosphere/1 -> Demux/1
  Demux/4 -> Divide/1
  rho0/1 -> Divide/2
  Divide/1 -> Exp/1
  n/1 -> Exp/2
  Divide1/1 -> Thrust/1
  Wind_Vel/1 -> Divide1/2
  Dot Product2/1 -> Dot Product/1
  Power - W (315hp)/1 -> Dot Product2/2
  eta_p/1 -> Dot Product2/1
  Demux/1 -> Terminator/1
  Demux/2 -> Terminator1/1
  Demux/3 -> Terminator2/1
  Dot Product/1 -> Divide1/1

== system SIM_3DoF/Subsystem ==
  states : Inport
  Demux : Demux  Outputs=6
  Gain : Gain  Gain=-1
  ISA Atmosphere Model : aerolibatmos2/ISA Atmosphere Model  useExtended=off  action=Warning  custom=off  viscosityOut=off  g=9.80665  gamma=1.4  R=287.0531  L=0.0065  h_trop=11000  h_strat=20000  rho0=1.225  P0=101325  T0=288.15  h0=0  S=110.4  Tref=273.15  muref=1.716e-5
  Mux : Mux
  Terminator{,1..4} (5 alike) : Terminator
  Atmosphere : Outport
  wires:
  ISA Atmosphere Model/1 -> Mux/1
  ISA Atmosphere Model/2 -> Mux/2
  ISA Atmosphere Model/3 -> Mux/3
  Mux/1 -> Atmosphere/1
  states/1 -> Demux/1
  Demux/6 -> Terminator/1
  Demux/5 -> Terminator1/1
  Demux/4 -> Terminator2/1
  Demux/1 -> Terminator3/1
  Demux/3 -> Terminator4/1
  ISA Atmosphere Model/4 -> Mux/4
  Demux/2 -> Gain/1
  Gain/1 -> ISA Atmosphere Model/1

== system SIM_3DoF/Subsystem1 ==
  states : Inport
  Demux : Demux  Outputs=6
  Gain : Gain  Gain=-1
  ISA Atmosphere Model : aerolibatmos2/ISA Atmosphere Model  useExtended=off  action=Warning  custom=off  viscosityOut=off  g=9.80665  gamma=1.4  R=287.0531  L=0.0065  h_trop=11000  h_strat=20000  rho0=1.225  P0=101325  T0=288.15  h0=0  S=110.4  Tref=273.15  muref=1.716e-5
  Mux : Mux
  Terminator{,1..4} (5 alike) : Terminator
  Atmosphere : Outport
  Height : Outport  Port=2
  wires:
  ISA Atmosphere Model/1 -> Mux/1
  ISA Atmosphere Model/2 -> Mux/2
  ISA Atmosphere Model/3 -> Mux/3
  Mux/1 -> Atmosphere/1
  states/1 -> Demux/1
  Demux/6 -> Terminator/1
  Demux/5 -> Terminator1/1
  Demux/4 -> Terminator2/1
  Demux/1 -> Terminator3/1
  Demux/3 -> Terminator4/1
  ISA Atmosphere Model/4 -> Mux/4
  Demux/2 -> Gain/1
  Gain/1 -> Height/1, ISA Atmosphere Model/1

== system SIM_3DoF/Subsystem2 ==
  states1 : Inport
  h : Inport  Port=2
  Add : Sum  Inputs=+-
  Constant1 : Constant  Value=states_init
  Demux1 : Demux  Outputs=6
  Demux2 : Demux  Outputs=6
  Minus : Sum  Inputs=-+
  Terminator{,1..5,8..9} (8 alike) : Terminator
  Height : Outport
  Theta : Outport  Port=2
  X Velocity : Outport  Port=3
  wires:
  Constant1/1 -> Demux2/1
  Demux1/3 -> Terminator4/1
  Demux1/4 -> Terminator2/1
  Demux1/1 -> Terminator3/1
  Demux2/6 -> Terminator9/1
  Demux1/2 -> Minus/2  "y"
  states1/1 -> Demux1/1
  Demux1/6 -> Terminator/1
  Demux1/5 -> Terminator1/1
  Demux2/2 -> Add/1, Minus/1  "y_init"
  Minus/1 -> Add/2
  Add/1 -> Height/1  "Height"
  Demux2/3 -> Theta/1
  Demux2/1 -> Terminator5/1
  Demux2/5 -> Terminator8/1
  Demux2/4 -> X Velocity/1

== system SIM_3DoF/Throttle Control ==
  Throttle : Inport
  Add1 : Sum
  Constant : Constant  Value=throttle
  Power Setting : Outport
  wires:
  Throttle/1 -> Add1/1
  Constant/1 -> Add1/2
  Add1/1 -> Power Setting/1

== system SIM_3DoF/Throttle Control1 ==
  Throttle : Inport
  Throttle from controller : Inport  Port=2
  Add1 : Sum
  Constant : Constant  Value=throttle
  Manual Switch : ManualSwitch
  Power Setting : Outport
  wires:
  Throttle/1 -> Add1/1
  Constant/1 -> Add1/2
  Add1/1 -> Manual Switch/1
  Throttle from controller/1 -> Manual Switch/2
  Manual Switch/1 -> Power Setting/1

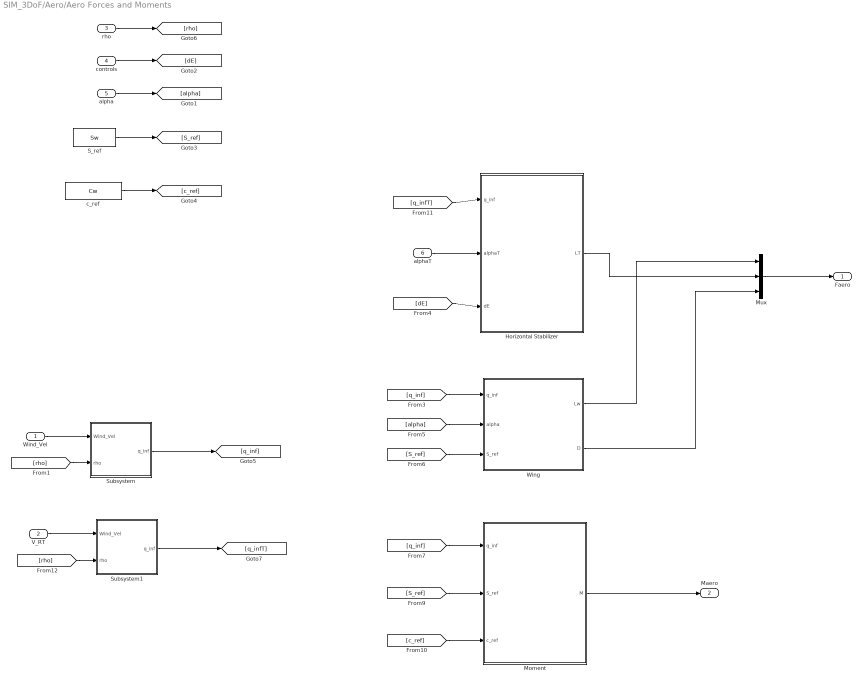
== system SIM_3DoF/Aero/Aero Forces and Moments ==
  Wind_Vel : Inport
  V_RT : Inport  Port=2
  rho : Inport  Port=3
  controls : Inport  Port=4
  alpha : Inport  Port=5
  alphaT : Inport  Port=6
  Horizontal Stabilizer : Subsystem
  Moment : Subsystem
  Mux : Mux  Inputs=3
  S_ref : Constant  Value=Sw
  Subsystem : Subsystem
  Subsystem1 : Subsystem
  Wing : Subsystem
  c_ref : Constant  Value=Cw
  Faero : Outport
  Maero : Outport  Port=2
  wires:
  Mux/1 -> Faero/1
  Wind_Vel/1 -> Subsystem/1(Wind_Vel)
  Horizontal Stabilizer/1(LT) -> Mux/2
  Wing/1(Lw) -> Mux/1
  Wing/2(D) -> Mux/3
  Moment/1(M) -> Maero/1
  alphaT/1 -> Horizontal Stabilizer/2(alphaT)
  controls/1 -> [dE]
  [dE] -> Horizontal Stabilizer/3(dE)
  c_ref/1 -> [c_ref]
  S_ref/1 -> [S_ref]
  alpha/1 -> [alpha]
  Subsystem/1(q_inf) -> [q_inf]
  [q_infT] -> Horizontal Stabilizer/1(q_inf)
  [q_inf] -> Wing/1(q_inf)
  [alpha] -> Wing/2(alpha)
  [S_ref] -> Wing/3(S_ref)
  [c_ref] -> Moment/3(c_ref)
  [S_ref] -> Moment/2(S_ref)
  [q_inf] -> Moment/1(q_inf)
  rho/1 -> [rho]
  [rho] -> Subsystem/2(rho)
  [rho] -> Subsystem1/2(rho)
  Subsystem1/1(q_inf) -> [q_infT]
  V_RT/1 -> Subsystem1/1(Wind_Vel)

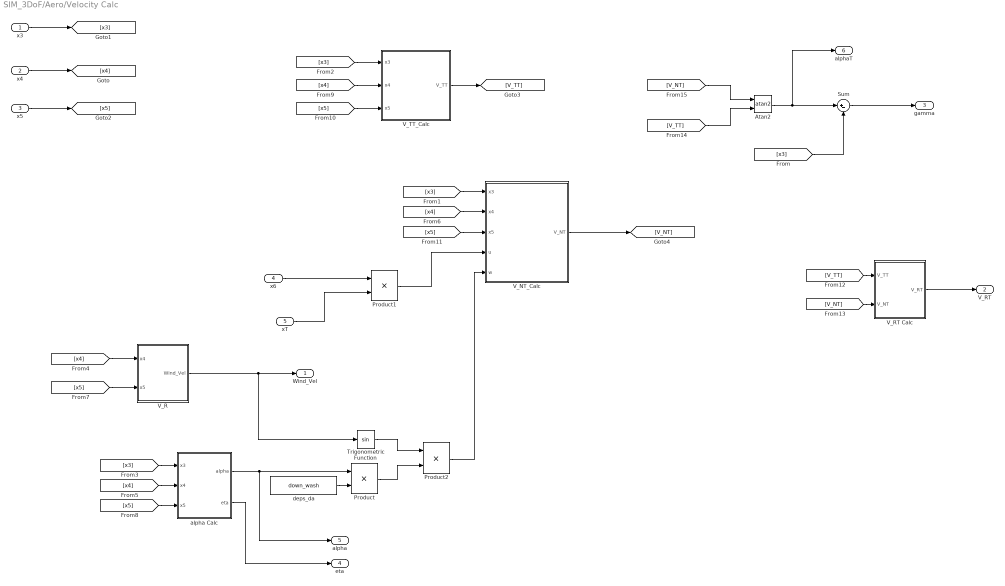
== system SIM_3DoF/Aero/Velocity Calc ==
  x3 : Inport
  x4 : Inport  Port=2
  x5 : Inport  Port=3
  x6 : Inport  Port=4
  xT : Inport  Port=5
  Atan2 : Trigonometry  Operator=atan2
  Product : Product
  Product1 : Product
  Product2 : Product
  Sum : Sum  Inputs=|+-
  Trigonometric Function : Trigonometry
  V_NT_Calc : Subsystem
  V_R : Subsystem
  V_RT Calc : Subsystem
  V_TT_Calc : Subsystem
  alpha Calc : Subsystem
  deps_da : Constant  Value=down_wash
  Wind_Vel : Outport
  V_RT : Outport  Port=2
  gamma : Outport  Port=3
  eta : Outport  Port=4
  alpha : Outport  Port=5
  alphaT : Outport  Port=6
  wires:
  V_R/1(Wind_Vel) -> Trigonometric Function/1, Wind_Vel/1
  x5/1 -> [x5]
  x4/1 -> [x4]
  x6/1 -> Product1/1
  deps_da/1 -> Product/2
  x3/1 -> [x3]
  Atan2/1 -> alphaT/1, Sum/1
  Sum/1 -> gamma/1
  alpha Calc/2(eta) -> eta/1
  xT/1 -> Product1/2
  [x3] -> Sum/2
  [x3] -> V_TT_Calc/1(x3)
  [x3] -> alpha Calc/1(x3)
  [x4] -> V_R/1(x4)
  [x4] -> alpha Calc/2(x4)
  [x5] -> V_R/2(x5)
  [x5] -> alpha Calc/3(x5)
  [x4] -> V_TT_Calc/2(x4)
  V_TT_Calc/1(V_TT) -> [V_TT]
  V_NT_Calc/1(V_NT) -> [V_NT]
  [V_TT] -> V_RT Calc/1(V_TT)
  [V_NT] -> V_RT Calc/2(V_NT)
  [V_NT] -> Atan2/1
  [V_TT] -> Atan2/2
  V_RT Calc/1(V_RT) -> V_RT/1
  [x5] -> V_TT_Calc/3(x5)
  [x5] -> V_NT_Calc/3(x5)
  alpha Calc/1(alpha) -> alpha/1, Product/1
  [x3] -> V_NT_Calc/1(x3)
  [x4] -> V_NT_Calc/2(x4)
  Product/1 -> Product2/2
  Trigonometric Function/1 -> Product2/1
  Product2/1 -> V_NT_Calc/5(w)
  Product1/1 -> V_NT_Calc/4(u)

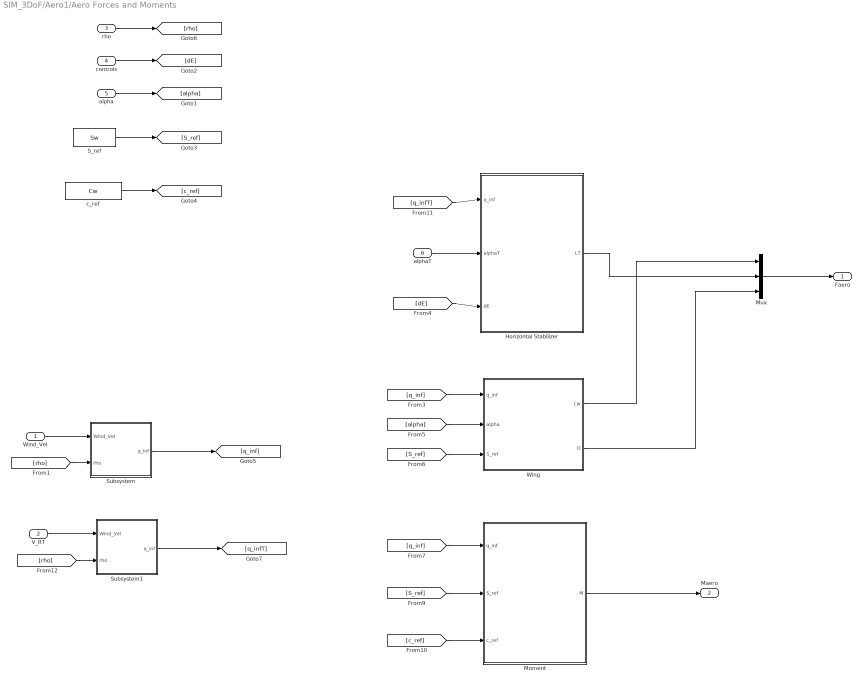
== system SIM_3DoF/Aero1/Aero Forces and Moments ==
  Wind_Vel : Inport
  V_RT : Inport  Port=2
  rho : Inport  Port=3
  controls : Inport  Port=4
  alpha : Inport  Port=5
  alphaT : Inport  Port=6
  Horizontal Stabilizer : Subsystem
  Moment : Subsystem
  Mux : Mux  Inputs=3
  S_ref : Constant  Value=Sw
  Subsystem : Subsystem
  Subsystem1 : Subsystem
  Wing : Subsystem
  c_ref : Constant  Value=Cw
  Faero : Outport
  Maero : Outport  Port=2
  wires:
  Mux/1 -> Faero/1
  Wind_Vel/1 -> Subsystem/1(Wind_Vel)
  Horizontal Stabilizer/1(LT) -> Mux/2
  Wing/1(Lw) -> Mux/1
  Wing/2(D) -> Mux/3
  Moment/1(M) -> Maero/1
  alphaT/1 -> Horizontal Stabilizer/2(alphaT)
  controls/1 -> [dE]
  [dE] -> Horizontal Stabilizer/3(dE)
  c_ref/1 -> [c_ref]
  S_ref/1 -> [S_ref]
  alpha/1 -> [alpha]
  Subsystem/1(q_inf) -> [q_inf]
  [q_infT] -> Horizontal Stabilizer/1(q_inf)
  [q_inf] -> Wing/1(q_inf)
  [alpha] -> Wing/2(alpha)
  [S_ref] -> Wing/3(S_ref)
  [c_ref] -> Moment/3(c_ref)
  [S_ref] -> Moment/2(S_ref)
  [q_inf] -> Moment/1(q_inf)
  rho/1 -> [rho]
  [rho] -> Subsystem/2(rho)
  [rho] -> Subsystem1/2(rho)
  Subsystem1/1(q_inf) -> [q_infT]
  V_RT/1 -> Subsystem1/1(Wind_Vel)

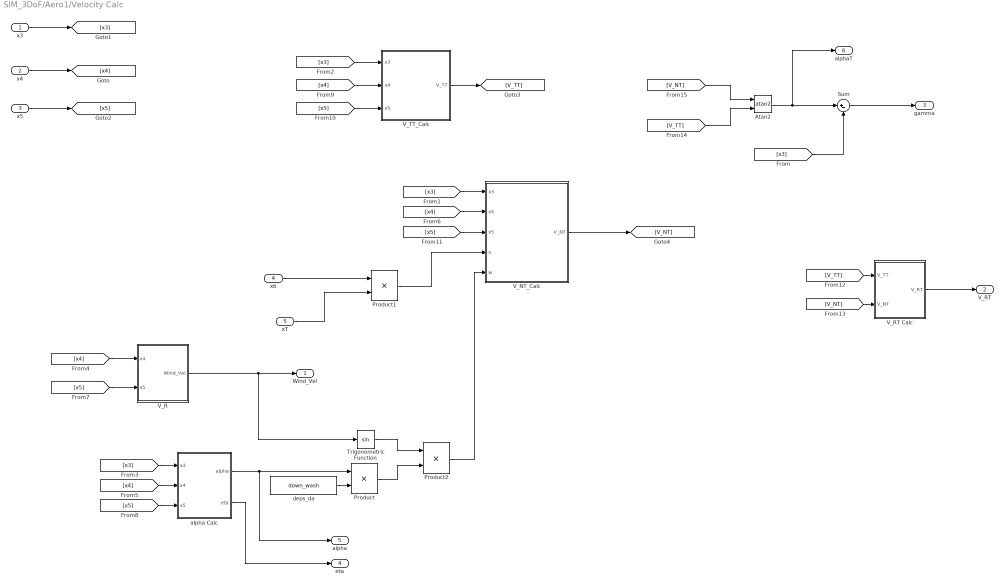
== system SIM_3DoF/Aero1/Velocity Calc ==
  x3 : Inport
  x4 : Inport  Port=2
  x5 : Inport  Port=3
  x6 : Inport  Port=4
  xT : Inport  Port=5
  Atan2 : Trigonometry  Operator=atan2
  Product : Product
  Product1 : Product
  Product2 : Product
  Sum : Sum  Inputs=|+-
  Trigonometric Function : Trigonometry
  V_NT_Calc : Subsystem
  V_R : Subsystem
  V_RT Calc : Subsystem
  V_TT_Calc : Subsystem
  alpha Calc : Subsystem
  deps_da : Constant  Value=down_wash
  Wind_Vel : Outport
  V_RT : Outport  Port=2
  gamma : Outport  Port=3
  eta : Outport  Port=4
  alpha : Outport  Port=5
  alphaT : Outport  Port=6
  wires:
  V_R/1(Wind_Vel) -> Trigonometric Function/1, Wind_Vel/1
  x5/1 -> [x5]
  x4/1 -> [x4]
  x6/1 -> Product1/1
  deps_da/1 -> Product/2
  x3/1 -> [x3]
  Atan2/1 -> alphaT/1, Sum/1
  Sum/1 -> gamma/1
  alpha Calc/2(eta) -> eta/1
  xT/1 -> Product1/2
  [x3] -> Sum/2
  [x3] -> V_TT_Calc/1(x3)
  [x3] -> alpha Calc/1(x3)
  [x4] -> V_R/1(x4)
  [x4] -> alpha Calc/2(x4)
  [x5] -> V_R/2(x5)
  [x5] -> alpha Calc/3(x5)
  [x4] -> V_TT_Calc/2(x4)
  V_TT_Calc/1(V_TT) -> [V_TT]
  V_NT_Calc/1(V_NT) -> [V_NT]
  [V_TT] -> V_RT Calc/1(V_TT)
  [V_NT] -> V_RT Calc/2(V_NT)
  [V_NT] -> Atan2/1
  [V_TT] -> Atan2/2
  V_RT Calc/1(V_RT) -> V_RT/1
  [x5] -> V_TT_Calc/3(x5)
  [x5] -> V_NT_Calc/3(x5)
  alpha Calc/1(alpha) -> alpha/1, Product/1
  [x3] -> V_NT_Calc/1(x3)
  [x4] -> V_NT_Calc/2(x4)
  Product/1 -> Product2/2
  Trigonometric Function/1 -> Product2/1
  Product2/1 -> V_NT_Calc/5(w)
  Product1/1 -> V_NT_Calc/4(u)

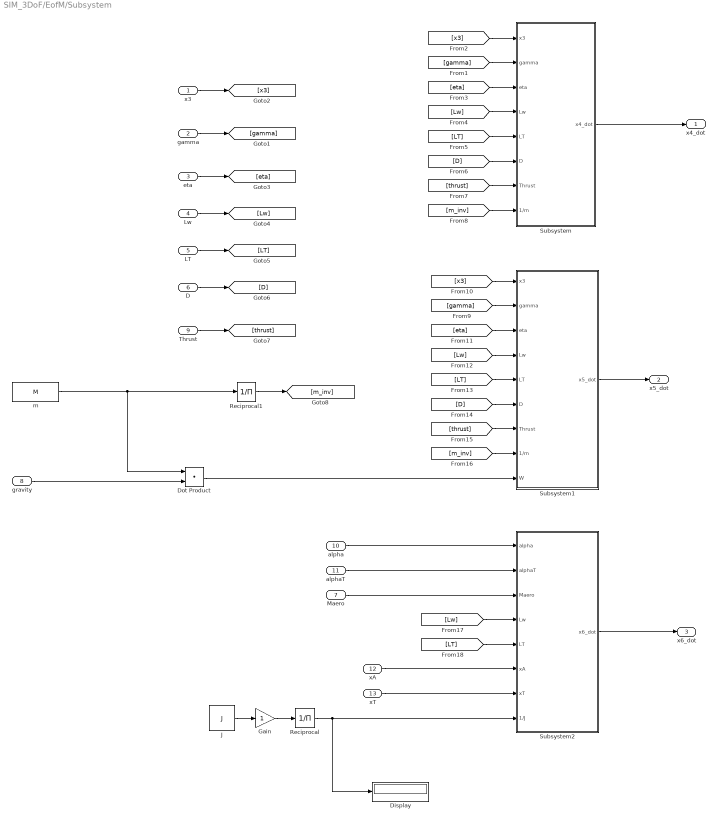
== system SIM_3DoF/EofM/Subsystem ==
  x3 : Inport
  gamma : Inport  Port=2
  eta : Inport  Port=3
  Lw : Inport  Port=4
  LT : Inport  Port=5
  D : Inport  Port=6
  Maero : Inport  Port=7
  gravity : Inport  Port=8
  Thrust : Inport  Port=9
  alpha : Inport  Port=10
  alphaT : Inport  Port=11
  "xA " : Inport  Port=12
  xT : Inport  Port=13
  Display : Display
  Dot Product : DotProduct  OutDataTypeStr=Inherit: Inherit via internal rule
  Gain : Gain
  J : Constant  Value=J
  Reciprocal : Product  Inputs=/
  Reciprocal1 : Product  Inputs=/
  Subsystem : Subsystem
  Subsystem1 : Subsystem
  Subsystem2 : Subsystem
  m : Constant  Value=M
  x4_dot : Outport
  x5_dot : Outport  Port=2
  x6_dot : Outport  Port=3
  wires:
  Reciprocal/1 -> Display/1, Subsystem2/8(1/J)
  Thrust/1 -> [thrust]
  Reciprocal1/1 -> [m_inv]
  Subsystem/1(x4_dot) -> x4_dot/1
  Subsystem1/1(x5_dot) -> x5_dot/1
  alpha/1 -> Subsystem2/1(alpha)
  alphaT/1 -> Subsystem2/2(alphaT)
  Maero/1 -> Subsystem2/3(Maero)
  "xA "/1 -> Subsystem2/6(xA)
  xT/1 -> Subsystem2/7(xT)
  Subsystem2/1(x6_dot) -> x6_dot/1
  x3/1 -> [x3]
  gamma/1 -> [gamma]
  eta/1 -> [eta]
  Lw/1 -> [Lw]
  D/1 -> [D]
  LT/1 -> [LT]
  [x3] -> Subsystem/1(x3)
  [gamma] -> Subsystem/2(gamma)
  [m_inv] -> Subsystem/8(1/m)
  [thrust] -> Subsystem/7(Thrust)
  [D] -> Subsystem/6(D)
  [LT] -> Subsystem/5(LT)
  [Lw] -> Subsystem/4(Lw)
  [eta] -> Subsystem/3(eta)
  [x3] -> Subsystem1/1(x3)
  [D] -> Subsystem1/6(D)
  [thrust] -> Subsystem1/7(Thrust)
  [Lw] -> Subsystem1/4(Lw)
  [gamma] -> Subsystem1/2(gamma)
  [eta] -> Subsystem1/3(eta)
  [m_inv] -> Subsystem1/8(1/m)
  [LT] -> Subsystem1/5(LT)
  m/1 -> Reciprocal1/1, Dot Product/1
  [Lw] -> Subsystem2/4(Lw)
  [LT] -> Subsystem2/5(LT)
  gravity/1 -> Dot Product/2
  Dot Product/1 -> Subsystem1/9(W)
  J/1 -> Gain/1
  Gain/1 -> Reciprocal/1

== system SIM_3DoF/EofM/Wind_Vel Calc ==
  x4 : Inport
  x5 : Inport  Port=2
  Sqrt : Sqrt
  Square : Math  Operator=square
  Square1 : Math  Operator=square
  Sum : Sum  Inputs=|++
  Wind_Vel : Outport
  wires:
  Sqrt/1 -> Wind_Vel/1
  x5/1 -> Square1/1
  Square1/1 -> Sum/2
  Sum/1 -> Sqrt/1
  x4/1 -> Square/1
  Square/1 -> Sum/1

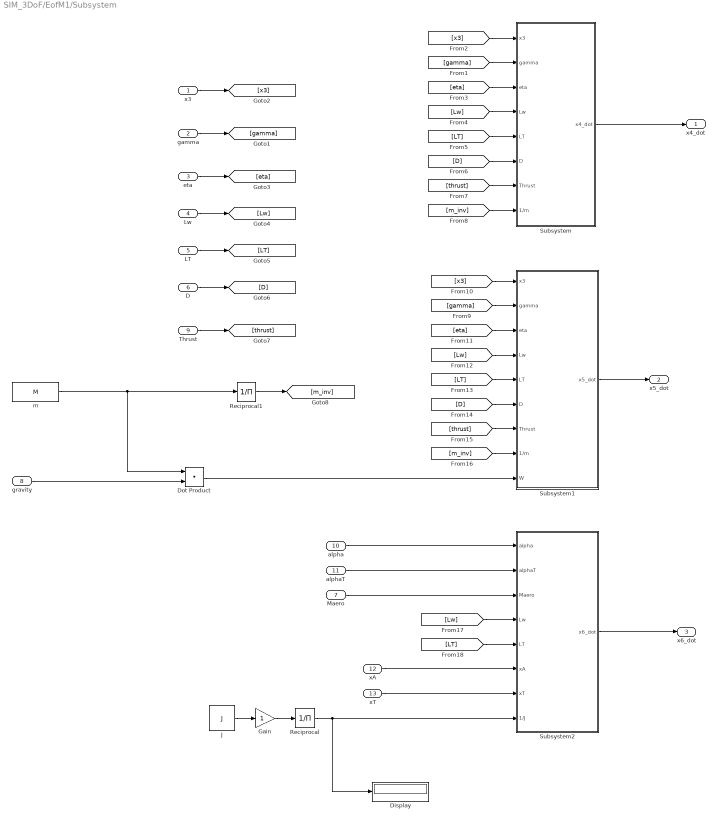
== system SIM_3DoF/EofM1/Subsystem ==
  x3 : Inport
  gamma : Inport  Port=2
  eta : Inport  Port=3
  Lw : Inport  Port=4
  LT : Inport  Port=5
  D : Inport  Port=6
  Maero : Inport  Port=7
  gravity : Inport  Port=8
  Thrust : Inport  Port=9
  alpha : Inport  Port=10
  alphaT : Inport  Port=11
  "xA " : Inport  Port=12
  xT : Inport  Port=13
  Display : Display
  Dot Product : DotProduct  OutDataTypeStr=Inherit: Inherit via internal rule
  Gain : Gain
  J : Constant  Value=J
  Reciprocal : Product  Inputs=/
  Reciprocal1 : Product  Inputs=/
  Subsystem : Subsystem
  Subsystem1 : Subsystem
  Subsystem2 : Subsystem
  m : Constant  Value=M
  x4_dot : Outport
  x5_dot : Outport  Port=2
  x6_dot : Outport  Port=3
  wires:
  Reciprocal/1 -> Display/1, Subsystem2/8(1/J)
  Thrust/1 -> [thrust]
  Reciprocal1/1 -> [m_inv]
  Subsystem/1(x4_dot) -> x4_dot/1
  Subsystem1/1(x5_dot) -> x5_dot/1
  alpha/1 -> Subsystem2/1(alpha)
  alphaT/1 -> Subsystem2/2(alphaT)
  Maero/1 -> Subsystem2/3(Maero)
  "xA "/1 -> Subsystem2/6(xA)
  xT/1 -> Subsystem2/7(xT)
  Subsystem2/1(x6_dot) -> x6_dot/1
  x3/1 -> [x3]
  gamma/1 -> [gamma]
  eta/1 -> [eta]
  Lw/1 -> [Lw]
  D/1 -> [D]
  LT/1 -> [LT]
  [x3] -> Subsystem/1(x3)
  [gamma] -> Subsystem/2(gamma)
  [m_inv] -> Subsystem/8(1/m)
  [thrust] -> Subsystem/7(Thrust)
  [D] -> Subsystem/6(D)
  [LT] -> Subsystem/5(LT)
  [Lw] -> Subsystem/4(Lw)
  [eta] -> Subsystem/3(eta)
  [x3] -> Subsystem1/1(x3)
  [D] -> Subsystem1/6(D)
  [thrust] -> Subsystem1/7(Thrust)
  [Lw] -> Subsystem1/4(Lw)
  [gamma] -> Subsystem1/2(gamma)
  [eta] -> Subsystem1/3(eta)
  [m_inv] -> Subsystem1/8(1/m)
  [LT] -> Subsystem1/5(LT)
  m/1 -> Reciprocal1/1, Dot Product/1
  [Lw] -> Subsystem2/4(Lw)
  [LT] -> Subsystem2/5(LT)
  gravity/1 -> Dot Product/2
  Dot Product/1 -> Subsystem1/9(W)
  J/1 -> Gain/1
  Gain/1 -> Reciprocal/1

== system SIM_3DoF/EofM1/Wind_Vel Calc ==
  x4 : Inport
  x5 : Inport  Port=2
  Sqrt : Sqrt
  Square : Math  Operator=square
  Square1 : Math  Operator=square
  Sum : Sum  Inputs=|++
  Wind_Vel : Outport
  wires:
  Sqrt/1 -> Wind_Vel/1
  x5/1 -> Square1/1
  Square1/1 -> Sum/2
  Sum/1 -> Sqrt/1
  x4/1 -> Square/1
  Square/1 -> Sum/1

== system SIM_3DoF/Aero/Aero Forces and Moments/Horizontal Stabilizer ==
  q_inf : Inport
  alphaT : Inport  Port=2
  dE : Inport  Port=3
  " " : DotProduct  OutDataTypeStr=Inherit: Inherit via internal rule
  Constant1 : Constant  Value=CLEH_alpha
  Constant2 : Constant  Value=CL_elev
  Dot Product : DotProduct  OutDataTypeStr=Inherit: Inherit via internal rule
  Dot Product1 : DotProduct  OutDataTypeStr=Inherit: Inherit via internal rule
  Dot Product2 : DotProduct  OutDataTypeStr=Inherit: Inherit via internal rule
  Sh : Constant  Value=Sh
  Sum : Sum  Inputs=|++
  LT : Outport
  wires:
  " "/1 -> LT/1
  Constant2/1 -> Dot Product/2
  dE/1 -> Dot Product/1
  Constant1/1 -> Dot Product1/1
  Dot Product1/1 -> Sum/2
  q_inf/1 -> Dot Product2/1
  Sum/1 -> Dot Product2/2
  Dot Product2/1 -> " "/1
  alphaT/1 -> Dot Product1/2
  Dot Product/1 -> Sum/1
  Sh/1 -> " "/2

== system SIM_3DoF/Aero/Aero Forces and Moments/Moment ==
  q_inf : Inport
  S_ref : Inport  Port=2
  c_ref : Inport  Port=3
  CM0 : Constant  Value=Cm_zero
  Dot Product1 : DotProduct  OutDataTypeStr=Inherit: Inherit via internal rule
  Dot Product2 : DotProduct  OutDataTypeStr=Inherit: Inherit via internal rule
  Dot Product6 : DotProduct  OutDataTypeStr=Inherit: Inherit via internal rule
  M : Outport
  wires:
  Dot Product1/1 -> Dot Product2/1
  q_inf/1 -> Dot Product1/1
  c_ref/1 -> Dot Product6/2
  S_ref/1 -> Dot Product2/2
  Dot Product6/1 -> M/1
  Dot Product2/1 -> Dot Product6/1
  CM0/1 -> Dot Product1/2

== system SIM_3DoF/Aero/Aero Forces and Moments/Subsystem ==
  Wind_Vel : Inport
  rho : Inport  Port=2
  Constant : Constant  Value=0.5
  Product : Product  Inputs=3
  Square : Math  Operator=square
  q_inf : Outport
  wires:
  Wind_Vel/1 -> Square/1
  Square/1 -> Product/1
  rho/1 -> Product/2
  Constant/1 -> Product/3
  Product/1 -> q_inf/1

== system SIM_3DoF/Aero/Aero Forces and Moments/Subsystem1 ==
  Wind_Vel : Inport
  rho : Inport  Port=2
  Constant : Constant  Value=0.5
  Product : Product  Inputs=3
  Square : Math  Operator=square
  q_inf : Outport
  wires:
  Wind_Vel/1 -> Square/1
  Square/1 -> Product/1
  rho/1 -> Product/2
  Constant/1 -> Product/3
  Product/1 -> q_inf/1

== system SIM_3DoF/Aero/Aero Forces and Moments/Wing ==
  q_inf : Inport
  alpha : Inport  Port=2
  S_ref : Inport  Port=3
  1-D Lookup Table1 : Lookup_n-D  NumberOfTableDimensions=1  BreakpointsForDimension1=CD_alpha(:, 1)  Table=CD_alpha(:, 2)  InternalRulePriority=Speed  RndMeth=Simplest
  CLw0 : Constant  Value=CL_zero
  Gain : Gain  Gain=CL_alpha
  Plus : Sum
  Product : Product  Inputs=3
  Product1 : Product  Inputs=3
  Lw : Outport
  D : Outport  Port=2
  wires:
  Product/1 -> Lw/1
  CLw0/1 -> Plus/1
  Plus/1 -> Product/1
  q_inf/1 -> [q_inf]
  S_ref/1 -> [S_ref]
  [S_ref] -> Product/3
  Gain/1 -> Plus/2
  alpha/1 -> [alpha]
  [alpha] -> 1-D Lookup Table1/1
  [q_inf] -> Product/2
  Product1/1 -> D/1
  [S_ref] -> Product1/3
  [q_inf] -> Product1/2
  [alpha] -> Gain/1
  1-D Lookup Table1/1 -> Product1/1

== system SIM_3DoF/Aero/Velocity Calc/V_NT_Calc ==
  x3 : Inport
  x4 : Inport  Port=2
  x5 : Inport  Port=3
  u : Inport  Port=4
  w : Inport  Port=5
  Cos : Trigonometry
  Dot Product : DotProduct  OutDataTypeStr=Inherit: Inherit via internal rule
  Dot Product1 : DotProduct  OutDataTypeStr=Inherit: Inherit via internal rule
  Sin : Trigonometry  Operator=cos
  Subtract : Sum
  Sum2 : Sum  Inputs=|++
  Sum3 : Sum  Inputs=|+-
  V_NT : Outport
  wires:
  u/1 -> Sum2/2
  w/1 -> Sum3/2
  Sum2/1 -> Sum3/1
  Sum3/1 -> V_NT/1
  x4/1 -> Dot Product/2
  Dot Product/1 -> Subtract/1
  x5/1 -> Dot Product1/2
  x3/1 -> Sin/1, Cos/1
  Dot Product1/1 -> Subtract/2
  Sin/1 -> Dot Product1/1
  Cos/1 -> Dot Product/1
  Subtract/1 -> Sum2/1

== system SIM_3DoF/Aero/Velocity Calc/V_R ==
  x4 : Inport
  x5 : Inport  Port=2
  Sqrt : Sqrt
  Square : Math  Operator=square
  Square1 : Math  Operator=square
  Sum : Sum  Inputs=|++
  Wind_Vel : Outport
  wires:
  Sqrt/1 -> Wind_Vel/1
  x5/1 -> Square1/1
  Square1/1 -> Sum/2
  Sum/1 -> Sqrt/1
  x4/1 -> Square/1
  Square/1 -> Sum/1

== system SIM_3DoF/Aero/Velocity Calc/V_RT Calc ==
  V_TT : Inport
  V_NT : Inport  Port=2
  Sqrt : Sqrt
  Square : Math  Operator=square
  Square1 : Math  Operator=square
  Sum : Sum  Inputs=|++
  V_RT : Outport
  wires:
  V_TT/1 -> Square/1
  Sqrt/1 -> V_RT/1
  Square/1 -> Sum/1
  Sum/1 -> Sqrt/1
  V_NT/1 -> Square1/1
  Square1/1 -> Sum/2

== system SIM_3DoF/Aero/Velocity Calc/V_TT_Calc ==
  x3 : Inport
  x4 : Inport  Port=2
  x5 : Inport  Port=3
  Cos : Trigonometry  Operator=cos
  Dot Product : DotProduct  OutDataTypeStr=Inherit: Inherit via internal rule
  Dot Product1 : DotProduct  OutDataTypeStr=Inherit: Inherit via internal rule
  Sin : Trigonometry
  Subtract : Sum  Inputs=+-
  V_TT : Outport
  wires:
  Subtract/1 -> V_TT/1
  x3/1 -> Sin/1, Cos/1
  Cos/1 -> Dot Product/1
  x4/1 -> Dot Product/2
  Sin/1 -> Dot Product1/1
  x5/1 -> Dot Product1/2
  Dot Product/1 -> Subtract/1
  Dot Product1/1 -> Subtract/2

== system SIM_3DoF/Aero/Velocity Calc/alpha Calc ==
  x3 : Inport
  x4 : Inport  Port=2
  x5 : Inport  Port=3
  Atan2 : Trigonometry  Operator=atan2
  Sum : Sum  Inputs=|++
  alpha : Outport
  eta : Outport  Port=2
  wires:
  x3/1 -> Sum/2
  Atan2/1 -> Sum/1, eta/1
  x5/1 -> Atan2/1
  x4/1 -> Atan2/2
  Sum/1 -> alpha/1

== system SIM_3DoF/Aero1/Aero Forces and Moments/Horizontal Stabilizer ==
  q_inf : Inport
  alphaT : Inport  Port=2
  dE : Inport  Port=3
  " " : DotProduct  OutDataTypeStr=Inherit: Inherit via internal rule
  Constant1 : Constant  Value=CLEH_alpha
  Constant2 : Constant  Value=CL_elev
  Dot Product : DotProduct  OutDataTypeStr=Inherit: Inherit via internal rule
  Dot Product1 : DotProduct  OutDataTypeStr=Inherit: Inherit via internal rule
  Dot Product2 : DotProduct  OutDataTypeStr=Inherit: Inherit via internal rule
  Sh : Constant  Value=Sh
  Sum : Sum  Inputs=|++
  LT : Outport
  wires:
  " "/1 -> LT/1
  Constant2/1 -> Dot Product/2
  dE/1 -> Dot Product/1
  Constant1/1 -> Dot Product1/1
  Dot Product1/1 -> Sum/2
  q_inf/1 -> Dot Product2/1
  Sum/1 -> Dot Product2/2
  Dot Product2/1 -> " "/1
  alphaT/1 -> Dot Product1/2
  Dot Product/1 -> Sum/1
  Sh/1 -> " "/2

== system SIM_3DoF/Aero1/Aero Forces and Moments/Moment ==
  q_inf : Inport
  S_ref : Inport  Port=2
  c_ref : Inport  Port=3
  CM0 : Constant  Value=Cm_zero
  Dot Product1 : DotProduct  OutDataTypeStr=Inherit: Inherit via internal rule
  Dot Product2 : DotProduct  OutDataTypeStr=Inherit: Inherit via internal rule
  Dot Product6 : DotProduct  OutDataTypeStr=Inherit: Inherit via internal rule
  M : Outport
  wires:
  Dot Product1/1 -> Dot Product2/1
  q_inf/1 -> Dot Product1/1
  c_ref/1 -> Dot Product6/2
  S_ref/1 -> Dot Product2/2
  Dot Product6/1 -> M/1
  Dot Product2/1 -> Dot Product6/1
  CM0/1 -> Dot Product1/2

== system SIM_3DoF/Aero1/Aero Forces and Moments/Subsystem ==
  Wind_Vel : Inport
  rho : Inport  Port=2
  Constant : Constant  Value=0.5
  Product : Product  Inputs=3
  Square : Math  Operator=square
  q_inf : Outport
  wires:
  Wind_Vel/1 -> Square/1
  Square/1 -> Product/1
  rho/1 -> Product/2
  Constant/1 -> Product/3
  Product/1 -> q_inf/1

== system SIM_3DoF/Aero1/Aero Forces and Moments/Subsystem1 ==
  Wind_Vel : Inport
  rho : Inport  Port=2
  Constant : Constant  Value=0.5
  Product : Product  Inputs=3
  Square : Math  Operator=square
  q_inf : Outport
  wires:
  Wind_Vel/1 -> Square/1
  Square/1 -> Product/1
  rho/1 -> Product/2
  Constant/1 -> Product/3
  Product/1 -> q_inf/1

== system SIM_3DoF/Aero1/Aero Forces and Moments/Wing ==
  q_inf : Inport
  alpha : Inport  Port=2
  S_ref : Inport  Port=3
  1-D Lookup Table1 : Lookup_n-D  NumberOfTableDimensions=1  BreakpointsForDimension1=CD_alpha(:, 1)  Table=CD_alpha(:, 2)  InternalRulePriority=Speed  RndMeth=Simplest
  CLw0 : Constant  Value=CL_zero
  Gain : Gain  Gain=CL_alpha
  Plus : Sum
  Product : Product  Inputs=3
  Product1 : Product  Inputs=3
  Lw : Outport
  D : Outport  Port=2
  wires:
  Product/1 -> Lw/1
  CLw0/1 -> Plus/1
  Plus/1 -> Product/1
  q_inf/1 -> [q_inf]
  S_ref/1 -> [S_ref]
  [S_ref] -> Product/3
  Gain/1 -> Plus/2
  alpha/1 -> [alpha]
  [alpha] -> 1-D Lookup Table1/1
  [q_inf] -> Product/2
  Product1/1 -> D/1
  [S_ref] -> Product1/3
  [q_inf] -> Product1/2
  [alpha] -> Gain/1
  1-D Lookup Table1/1 -> Product1/1

== system SIM_3DoF/Aero1/Velocity Calc/V_NT_Calc ==
  x3 : Inport
  x4 : Inport  Port=2
  x5 : Inport  Port=3
  u : Inport  Port=4
  w : Inport  Port=5
  Cos : Trigonometry
  Dot Product : DotProduct  OutDataTypeStr=Inherit: Inherit via internal rule
  Dot Product1 : DotProduct  OutDataTypeStr=Inherit: Inherit via internal rule
  Sin : Trigonometry  Operator=cos
  Subtract : Sum
  Sum2 : Sum  Inputs=|++
  Sum3 : Sum  Inputs=|+-
  V_NT : Outport
  wires:
  u/1 -> Sum2/2
  w/1 -> Sum3/2
  Sum2/1 -> Sum3/1
  Sum3/1 -> V_NT/1
  x4/1 -> Dot Product/2
  Dot Product/1 -> Subtract/1
  x5/1 -> Dot Product1/2
  x3/1 -> Sin/1, Cos/1
  Dot Product1/1 -> Subtract/2
  Sin/1 -> Dot Product1/1
  Cos/1 -> Dot Product/1
  Subtract/1 -> Sum2/1

== system SIM_3DoF/Aero1/Velocity Calc/V_R ==
  x4 : Inport
  x5 : Inport  Port=2
  Sqrt : Sqrt
  Square : Math  Operator=square
  Square1 : Math  Operator=square
  Sum : Sum  Inputs=|++
  Wind_Vel : Outport
  wires:
  Sqrt/1 -> Wind_Vel/1
  x5/1 -> Square1/1
  Square1/1 -> Sum/2
  Sum/1 -> Sqrt/1
  x4/1 -> Square/1
  Square/1 -> Sum/1

== system SIM_3DoF/Aero1/Velocity Calc/V_RT Calc ==
  V_TT : Inport
  V_NT : Inport  Port=2
  Sqrt : Sqrt
  Square : Math  Operator=square
  Square1 : Math  Operator=square
  Sum : Sum  Inputs=|++
  V_RT : Outport
  wires:
  V_TT/1 -> Square/1
  Sqrt/1 -> V_RT/1
  Square/1 -> Sum/1
  Sum/1 -> Sqrt/1
  V_NT/1 -> Square1/1
  Square1/1 -> Sum/2
